simulink library "dotFinder_ul"  (R2018b)
settings: Solver=VariableStepAuto  StartTime=0.0  StopTime=10.0  RelTol=1e-3
libraries: simulink x2
settings Model: Creator=mcobb  LastModifiedBy=MAE-NCSUCORE
settings DebuggingCC: LibraryContextMissingDiagnostic=none
settings SFSimCC: SimUseLocalCustomCode=off
settings RTWCC: RTWUseLocalCustomCode=off

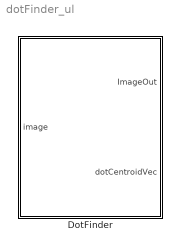
== system dotFinder_ul ==
  DotFinder : Subsystem  mask{ROIPositionHoldEnable=on, ROIPositionHoldCoordinates=[500 500], ROIDimVec_px=[30 90], ROIHalfDimVec_px=[15 45], ROISplitDims_px=[1 15 ; 1 90 ; 16 14 ; 1 90], DotOrientation=Vertical, OverlayOutput=on, ImageDimensions=[765 998], CrosshairPixelWidth_px=1}
      mask prompts: ROIPositionHoldEnable "Hold Position Enable"; ROIPositionHoldCoordinates "Hold Position Coordinates  [rows cols]  (pixels)"; ROIDimVec_px "Dimensions [rows cols]  (pixels)"; ROIHalfDimVec_px "Half Dims  [rows cols]  (pixels)"; ROISplitDims_px "Split Dims [rows cols]  (pixels)"; DotOrientation "Dot Orientation"; OverlayOutput "Draw Output Overlay"; ImageDimensions "Image Dimensions [rows cols] pixels"; CrosshairPixelWidth_px "Crosshair Width (pixels)"
      mask init:
      | dotFinder_init
      mask TypeOptions DotOrientation: Horizontal | Vertical
      mask DialogControl ParameterGroupVar Prompt: Region Of Interest (ROI) Parameters
      mask DialogControl Container3 Prompt: Other Parameters

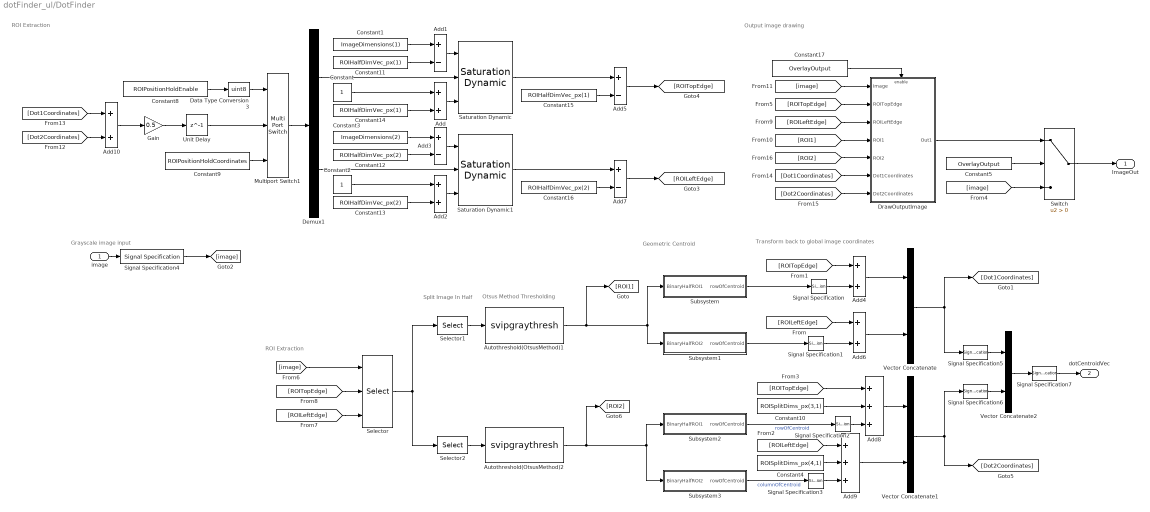
== system dotFinder_ul/DotFinder ==
  note: Transform back to global image coordinates
  note: Geometric Centroid
  note: Otsus Method Thresholding
  note: Split Image
      | In Half
  note: ROI Extraction
  note: Output image drawing
  note: ROI Extraction
  note: Grayscale image input
  image : Inport
  Add{,2,4,6,10} (5 alike) : Sum
  Add{1,3,5,7} (4 alike) : Sum  Inputs=+-
  Add8 : Sum  Inputs=+++
  Add9 : Sum  Inputs=+++
  Autothreshold(OtsusMethod)1 : S-Function  DialogController=vipDDGCreate  FunctionName=svipgraythresh  Parameters=operator, userDefinedRange, umin, umax, threshOut, effMetricOut, outOfRngOpt, scaleThreshold, scaleFactor, P1Mode, P1WordLength, P1FracLength, A1Mode, A1WordLength, A1FracLength, P2Mode, P2WordLength, P2FracLength, A2Mode, A2WordLength, A2FracLength, P3Mode, P3WordLength, P3FracLength, A3Mode, A3WordLength, A3FracLength, P4Mode, P4WordLength, P4FracLength, A4Mode, A4WordLength, A4FracLength, Q1Mode, Q1WordLength, Q1FracLength, EMMode, EMWordLength, EMFracLength, dtInfo.roundingMode, dtInfo.overflowMode  SFunctionDeploymentMode=off  EnableBusSupport=off  mask(Autothreshold){operator=>, threshOut=off, effMetricOut=off, userDefinedRange=off, umin=0, umax=255, outOfRngOpt=Ignore, scaleThreshold=off, scaleFactor=1, P1Mode=Specify word length, P1WordLength=32, P1FracLength=30, A1Mode=Same as Product 1, A1WordLength=32, A1FracLength=30, P2Mode=Specify word length, P2WordLength=32, P2FracLength=22, A2Mode=Same as Product 2, A2WordLength=32, A2FracLength=22, P3Mode=Specify word length, P3WordLength=32, P3FracLength=14, A3Mode=Same as Product 3, A3WordLength=32, A3FracLength=14, P4Mode=Binary point scaling, P4WordLength=32, P4FracLength=15, A4Mode=Same as Product 4, A4WordLength=16, A4FracLength=4, Q1Mode=Specify word length, Q1WordLength=32, Q1FracLength=16, EMMode=Specify word length, EMWordLength=16, EMFracLength=14, roundingMode=Floor, overflowMode=off, LockScale=off}
      mask prompts: operator "vision:masks:ThresholdingOperator"; threshOut "vision:masks:OutputThreshold"; effMetricOut "vision:masks:OutputEffectivenessMetric"; userDefinedRange "vision:masks:SpecifyDataRange"; umin "vision:masks:MinimumValueOfInput"; umax "vision:masks:MinimumValueOfInput"; outOfRngOpt "vision:masks:WhenDataRangeIsExceeded"; scaleThreshold "vision:masks:ScaleThreshold_MP"; scaleFactor "vision:masks:ThresholdScalingFactor"; P1Mode "P1:"; P1WordLength "P1 WL:"; P1FracLength "P1 FL:"; A1Mode "A1:"; A1WordLength "A1 WL:"; A1FracLength "A1 FL:"; P2Mode "P2:"; P2WordLength "P2 WL:"; P2FracLength "P2 FL:"; A2Mode "A2:"; A2WordLength "A2 WL:"; A2FracLength "A2 FL:"; P3Mode "P3:"; P3WordLength "P3 WL:"; P3FracLength "P3 FL:"; A3Mode "A3:"; A3WordLength "A3 WL:"; A3FracLength "A3 FL:"; P4Mode "P4:"; P4WordLength "P4 WL:"; P4FracLength "P4 FL:"; A4Mode "A4:"; A4WordLength "A4 WL:"; A4FracLength "A4 FL:"; Q1Mode "Q1:"; Q1WordLength "Q1 WL:"; Q1FracLength "Q1 FL:"; EMMode "EM:"; EMWordLength "EM WL:"; EMFracLength "EM FL:"; roundingMode "vision:masks:RoundIntegerCalculationsTowards"; overflowMode "vision:masks:RoundIntegerCalculationsTowards"; LockScale "vision:masks:LockScaling"
      mask help: vision:masks:AutoThresholdDescription
      mask init:
      | blk = gcbh;
      | 
      | dtInfo = dspGetFixptDataTypeInfo(blk,1);
      | 
      | effMetricOut_str = get_param(blk,'effMetricOut');
      | threshOut_str = get_param(blk,'threshOut');
      | if strcmp(effMetricOut_str,'off') && strcmp(threshOut_str,'off')
      | 	[so(1:3).port] = deal(1,1,1);
      | 	[so(1:3).txt] = deal('BW','BW','BW');
      | elseif strcmp(effMetricOut_str,'on') && strcmp(threshOut_str,'off')
      | 	[so(1:3).port] = deal(1,2,2);
      | 	[so(1:3).txt] = deal('BW','EMetric','EMetric');
      | elseif strcmp(effMetricOut_str,'off') && strcmp(threshOut_str,'on')
      | 	[so(1:3).port] = deal(1,2,2);
      | 	[so(1:3).txt] = deal('BW','Th','Th');
      | else
      | 	[so(1:3).port] = deal(1,2,3);
      | 	[so(1:3).txt] = deal('BW','Th','EMetric');
      | end
      mask Help: eval('visionblockhelp');
      mask TypeOptions operator: > | <=
      mask TypeOptions outOfRngOpt: vision:masks:Ignore | vision:masks:Saturate | vision:masks:WarnAndSaturate | vision:masks:Error
      mask TypeOptions P1Mode: Specify word length | Binary point scaling | Slope and bias scaling
      mask TypeOptions A1Mode: Same as Product 1 | Specify word length | Binary point scaling | Slope and bias scaling
      mask TypeOptions P2Mode: Specify word length | Binary point scaling | Slope and bias scaling
      mask TypeOptions A2Mode: Same as Product 2 | Specify word length | Binary point scaling | Slope and bias scaling
      mask TypeOptions P3Mode: Specify word length | Binary point scaling | Slope and bias scaling
      mask TypeOptions A3Mode: Same as Product 3 | Specify word length | Binary point scaling | Slope and bias scaling
      mask TypeOptions P4Mode: Same as input | Binary point scaling | Slope and bias scaling
      mask TypeOptions A4Mode: Same as Product 4 | Binary point scaling | Slope and bias scaling
      mask TypeOptions Q1Mode: Specify word length | Binary point scaling | Slope and bias scaling
      mask TypeOptions EMMode: Specify word length | Binary point scaling | Slope and bias scaling
      mask TypeOptions roundingMode: dspshared:FixptDialog:Ceiling_CB | dspshared:FixptDialog:Convergent_CB | dspshared:FixptDialog:Floor_CB | dspshared:FixptDialog:Nearest_CB | dspshared:FixptDialog:Round_CB | dspshared:FixptDialog:Simplest_CB | dspshared:FixptDialog:Zero_CB
      mask Display:
      | disp('Autothreshold');
      | port_label('input',1,'I');
      | port_label('output',so(1).port, so(1).txt);
      | port_label('output',so(2).port, so(2).txt);
      | port_label('output',so(3).port, so(3).txt);
  Autothreshold(OtsusMethod)2 : S-Function  DialogController=vipDDGCreate  FunctionName=svipgraythresh  Parameters=operator, userDefinedRange, umin, umax, threshOut, effMetricOut, outOfRngOpt, scaleThreshold, scaleFactor, P1Mode, P1WordLength, P1FracLength, A1Mode, A1WordLength, A1FracLength, P2Mode, P2WordLength, P2FracLength, A2Mode, A2WordLength, A2FracLength, P3Mode, P3WordLength, P3FracLength, A3Mode, A3WordLength, A3FracLength, P4Mode, P4WordLength, P4FracLength, A4Mode, A4WordLength, A4FracLength, Q1Mode, Q1WordLength, Q1FracLength, EMMode, EMWordLength, EMFracLength, dtInfo.roundingMode, dtInfo.overflowMode  SFunctionDeploymentMode=off  EnableBusSupport=off  mask(Autothreshold){operator=>, threshOut=off, effMetricOut=off, userDefinedRange=off, umin=0, umax=255, outOfRngOpt=Ignore, scaleThreshold=off, scaleFactor=1, P1Mode=Specify word length, P1WordLength=32, P1FracLength=30, A1Mode=Same as Product 1, A1WordLength=32, A1FracLength=30, P2Mode=Specify word length, P2WordLength=32, P2FracLength=22, A2Mode=Same as Product 2, A2WordLength=32, A2FracLength=22, P3Mode=Specify word length, P3WordLength=32, P3FracLength=14, A3Mode=Same as Product 3, A3WordLength=32, A3FracLength=14, P4Mode=Binary point scaling, P4WordLength=32, P4FracLength=15, A4Mode=Same as Product 4, A4WordLength=16, A4FracLength=4, Q1Mode=Specify word length, Q1WordLength=32, Q1FracLength=16, EMMode=Specify word length, EMWordLength=16, EMFracLength=14, roundingMode=Floor, overflowMode=off, LockScale=off}
      mask prompts: operator "vision:masks:ThresholdingOperator"; threshOut "vision:masks:OutputThreshold"; effMetricOut "vision:masks:OutputEffectivenessMetric"; userDefinedRange "vision:masks:SpecifyDataRange"; umin "vision:masks:MinimumValueOfInput"; umax "vision:masks:MinimumValueOfInput"; outOfRngOpt "vision:masks:WhenDataRangeIsExceeded"; scaleThreshold "vision:masks:ScaleThreshold_MP"; scaleFactor "vision:masks:ThresholdScalingFactor"; P1Mode "P1:"; P1WordLength "P1 WL:"; P1FracLength "P1 FL:"; A1Mode "A1:"; A1WordLength "A1 WL:"; A1FracLength "A1 FL:"; P2Mode "P2:"; P2WordLength "P2 WL:"; P2FracLength "P2 FL:"; A2Mode "A2:"; A2WordLength "A2 WL:"; A2FracLength "A2 FL:"; P3Mode "P3:"; P3WordLength "P3 WL:"; P3FracLength "P3 FL:"; A3Mode "A3:"; A3WordLength "A3 WL:"; A3FracLength "A3 FL:"; P4Mode "P4:"; P4WordLength "P4 WL:"; P4FracLength "P4 FL:"; A4Mode "A4:"; A4WordLength "A4 WL:"; A4FracLength "A4 FL:"; Q1Mode "Q1:"; Q1WordLength "Q1 WL:"; Q1FracLength "Q1 FL:"; EMMode "EM:"; EMWordLength "EM WL:"; EMFracLength "EM FL:"; roundingMode "vision:masks:RoundIntegerCalculationsTowards"; overflowMode "vision:masks:RoundIntegerCalculationsTowards"; LockScale "vision:masks:LockScaling"
      mask help: vision:masks:AutoThresholdDescription
      mask init: same as dotFinder_ul/DotFinder/Autothreshold(OtsusMethod)1
      mask Help: eval('visionblockhelp');
      mask TypeOptions operator: > | <=
      mask TypeOptions outOfRngOpt: vision:masks:Ignore | vision:masks:Saturate | vision:masks:WarnAndSaturate | vision:masks:Error
      mask TypeOptions P1Mode: Specify word length | Binary point scaling | Slope and bias scaling
      mask TypeOptions A1Mode: Same as Product 1 | Specify word length | Binary point scaling | Slope and bias scaling
      mask TypeOptions P2Mode: Specify word length | Binary point scaling | Slope and bias scaling
      mask TypeOptions A2Mode: Same as Product 2 | Specify word length | Binary point scaling | Slope and bias scaling
      mask TypeOptions P3Mode: Specify word length | Binary point scaling | Slope and bias scaling
      mask TypeOptions A3Mode: Same as Product 3 | Specify word length | Binary point scaling | Slope and bias scaling
      mask TypeOptions P4Mode: Same as input | Binary point scaling | Slope and bias scaling
      mask TypeOptions A4Mode: Same as Product 4 | Binary point scaling | Slope and bias scaling
      mask TypeOptions Q1Mode: Specify word length | Binary point scaling | Slope and bias scaling
      mask TypeOptions EMMode: Specify word length | Binary point scaling | Slope and bias scaling
      mask TypeOptions roundingMode: dspshared:FixptDialog:Ceiling_CB | dspshared:FixptDialog:Convergent_CB | dspshared:FixptDialog:Floor_CB | dspshared:FixptDialog:Nearest_CB | dspshared:FixptDialog:Round_CB | dspshared:FixptDialog:Simplest_CB | dspshared:FixptDialog:Zero_CB
      mask Display:
      | disp('Autothreshold');
      | port_label('input',1,'I');
      | port_label('output',so(1).port, so(1).txt);
      | port_label('output',so(2).port, so(2).txt);
      | port_label('output',so(3).port, so(3).txt);
  Constant : Constant
  Constant1 : Constant  Value=ImageDimensions(1)
  Constant10 : Constant  Value=ROISplitDims_px(3,1)
  Constant11 : Constant  Value=ROIHalfDimVec_px(1)
  Constant12 : Constant  Value=ROIHalfDimVec_px(2)
  Constant13 : Constant  Value=ROIHalfDimVec_px(2)
  Constant14 : Constant  Value=ROIHalfDimVec_px(1)
  Constant15 : Constant  Value=ROIHalfDimVec_px(1)
  Constant16 : Constant  Value=ROIHalfDimVec_px(2)
  Constant17 : Constant  Value=OverlayOutput
  Constant2 : Constant
  Constant3 : Constant  Value=ImageDimensions(2)
  Constant4 : Constant  Value=ROISplitDims_px(4,1)
  Constant5 : Constant  Value=OverlayOutput
  Constant8 : Constant  Value=ROIPositionHoldEnable
  Constant9 : Constant  Value=ROIPositionHoldCoordinates
  Data Type Conversion3 : DataTypeConversion  OutDataTypeStr=uint8
  Demux1 : Demux  Outputs=2
  DrawOutputImage : Subsystem
  Gain : Gain  Gain=0.5
  Multiport Switch1 : MultiPortSwitch  DataPortOrder=Zero-based contiguous  Inputs=2  zeroidx=on
  Saturation Dynamic : simulink/Discontinuities/Saturation Dynamic  OutMin=[]  OutMax=[]  OutDataTypeStr=Inherit: Same as second input  OutDataType=fixdt(1, 16)  OutScaling=2^-10  DoSatur=off
  Saturation Dynamic1 : simulink/Discontinuities/Saturation Dynamic  OutMin=[]  OutMax=[]  OutDataTypeStr=Inherit: Same as second input  OutDataType=fixdt(1, 16)  OutScaling=2^-10  DoSatur=off
  Selector : Selector  NumberOfDimensions=2  InputPortWidth=3  IndexOptions=Starting index (port),Starting index (port)  Indices=[1 3],1  OutputSizes=ROIDimVec_px(1),ROIDimVec_px(2)
  Selector1 : Selector  NumberOfDimensions=2  InputPortWidth=3  IndexOptions=Starting index (dialog),Starting index (dialog)  Indices=ROISplitDims_px(1,1),ROISplitDims_px(2,1)  OutputSizes=ROISplitDims_px(1,2),ROISplitDims_px(2,2)
  Selector2 : Selector  NumberOfDimensions=2  InputPortWidth=3  IndexOptions=Starting index (dialog),Starting index (dialog)  Indices=ROISplitDims_px(3,1),ROISplitDims_px(4,1)  OutputSizes=ROISplitDims_px(3,2),ROISplitDims_px(4,2)
  Signal Specification{,1..3} (4 alike) : SignalSpecification  Dimensions=1
  Signal Specification4 : SignalSpecification  Dimensions=ImageDimensions
  Signal Specification5 : SignalSpecification  Dimensions=[1 2]
  Signal Specification6 : SignalSpecification  Dimensions=[1 2]
  Signal Specification7 : SignalSpecification  Dimensions=[1 4]
  Subsystem : Subsystem
  Subsystem1 : Subsystem
  Subsystem2 : Subsystem
  Subsystem3 : Subsystem
  Switch : Switch  Criteria=u2 > Threshold
  Unit Delay : Delay  DelayLength=1  InitialCondition=ROIPositionHoldCoordinates
  Vector Concatenate : Concatenate
  Vector Concatenate1 : Concatenate
  Vector Concatenate2 : Concatenate  ConcatenateDimension=2
  ImageOut : Outport  PortDimensions=ImageDimensions
  dotCentroidVec : Outport  Port=2
  wires:
  Data Type Conversion3/1 -> Multiport Switch1/1
  Unit Delay/1 -> Multiport Switch1/2
  Multiport Switch1/1 -> Demux1/1
  Demux1/1 -> Saturation Dynamic/2
  Constant/1 -> Add/1
  Constant14/1 -> Add/2
  Constant1/1 -> Add1/1
  Constant11/1 -> Add1/2
  Constant12/1 -> Add3/2
  Constant3/1 -> Add3/1
  Constant13/1 -> Add2/2
  Constant2/1 -> Add2/1
  Demux1/2 -> Saturation Dynamic1/2
  Constant15/1 -> Add5/2
  Constant16/1 -> Add7/2
  [image] -> Selector/1
  Selector/1 -> Selector2/1, Selector1/1
  Constant8/1 -> Data Type Conversion3/1
  Constant9/1 -> Multiport Switch1/3
  Saturation Dynamic/1 -> Add5/1
  Saturation Dynamic1/1 -> Add7/1
  Add2/1 -> Saturation Dynamic1/3
  Add3/1 -> Saturation Dynamic1/1
  Add/1 -> Saturation Dynamic/3
  Add1/1 -> Saturation Dynamic/1
  Subsystem1/1(rowOfCentroid) -> Signal Specification1/1
  [ROITopEdge] -> Add4/1
  [ROILeftEdge] -> Add6/1
  Add4/1 -> Vector Concatenate/1
  Add6/1 -> Vector Concatenate/2
  Add9/1 -> Vector Concatenate1/2
  Add8/1 -> Vector Concatenate1/1
  [ROILeftEdge] -> Add9/1
  [ROITopEdge] -> Add8/1
  Subsystem3/1(rowOfCentroid) -> Signal Specification3/1  "columnOfCentroid"
  Subsystem2/1(rowOfCentroid) -> Signal Specification2/1  "rowOfCentroid"
  Selector2/1 -> Autothreshold(OtsusMethod)2/1
  Constant4/1 -> Add9/2
  Constant10/1 -> Add8/2
  Vector Concatenate1/1 -> Signal Specification6/1, [Dot2Coordinates]
  image/1 -> Signal Specification4/1
  Add7/1 -> [ROILeftEdge]
  Add5/1 -> [ROITopEdge]
  Constant17/1 -> DrawOutputImage/Enable
  DrawOutputImage/1(Out1) -> Switch/1
  [ROILeftEdge] -> Selector/3
  [ROITopEdge] -> Selector/2
  [ROITopEdge] -> DrawOutputImage/2(ROITopEdge)
  [ROILeftEdge] -> DrawOutputImage/3(ROILeftEdge)
  [ROI1] -> DrawOutputImage/4(ROI1)
  [image] -> Switch/3
  Constant5/1 -> Switch/2
  [image] -> DrawOutputImage/1(Image)
  Vector Concatenate/1 -> Signal Specification5/1, [Dot1Coordinates]
  [Dot2Coordinates] -> DrawOutputImage/7(Dot2Coordinates)
  [Dot1Coordinates] -> DrawOutputImage/6(Dot1Coordinates)
  Switch/1 -> ImageOut/1
  Selector1/1 -> Autothreshold(OtsusMethod)1/1
  Signal Specification/1 -> Add4/2
  Signal Specification1/1 -> Add6/2
  Signal Specification2/1 -> Add8/3
  Signal Specification3/1 -> Add9/3
  Signal Specification4/1 -> [image]
  Subsystem/1(rowOfCentroid) -> Signal Specification/1
  Autothreshold(OtsusMethod)2/1 -> [ROI2], Subsystem3/1(BinaryHalfROI2), Subsystem2/1(BinaryHalfROI1)
  Autothreshold(OtsusMethod)1/1 -> [ROI1], Subsystem1/1(BinaryHalfROI2), Subsystem/1(BinaryHalfROI1)
  [ROI2] -> DrawOutputImage/5(ROI2)
  Add10/1 -> Gain/1
  [Dot2Coordinates] -> Add10/2
  [Dot1Coordinates] -> Add10/1
  Gain/1 -> Unit Delay/1
  Vector Concatenate2/1 -> Signal Specification7/1
  Signal Specification5/1 -> Vector Concatenate2/1
  Signal Specification6/1 -> Vector Concatenate2/2
  Signal Specification7/1 -> dotCentroidVec/1

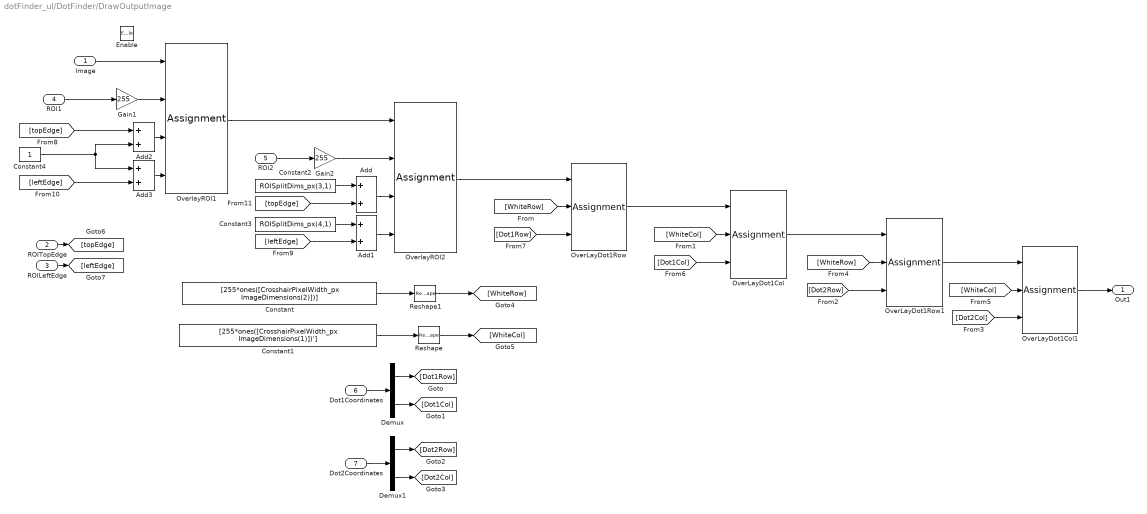
== system dotFinder_ul/DotFinder/DrawOutputImage ==
  Image : Inport
  ROITopEdge : Inport  Port=2
  ROILeftEdge : Inport  Port=3
  ROI1 : Inport  Port=4
  ROI2 : Inport  Port=5
  Dot1Coordinates : Inport  Port=6  PortDimensions=2
  Dot2Coordinates : Inport  Port=7  PortDimensions=2
  Enable : EnablePort
  Add{,1..3} (4 alike) : Sum
  Constant : Constant  Value=[255*ones([CrosshairPixelWidth_px ImageDimensions(2)])]  OutDataTypeStr=uint8
  Constant1 : Constant  Value=[255*ones([CrosshairPixelWidth_px ImageDimensions(1)])']  OutDataTypeStr=uint8
  Constant2 : Constant  Value=ROISplitDims_px(3,1)
  Constant3 : Constant  Value=ROISplitDims_px(4,1)
  Constant4 : Constant
  Demux : Demux  Outputs=2
  Demux1 : Demux  Outputs=2
  Gain1 : Gain  Gain=255  OutDataTypeStr=uint8
  Gain2 : Gain  Gain=255  OutDataTypeStr=uint8
  OverLayDot1Col : Assignment  NumberOfDimensions=2  DiagnosticForDimensions=Warning  IndexOptions=Assign all,Starting index (port)  Indices=1,1  OutputSizes=1,1
  OverLayDot1Col1 : Assignment  NumberOfDimensions=2  DiagnosticForDimensions=Warning  IndexOptions=Assign all,Starting index (port)  Indices=1,1  OutputSizes=1,1
  OverLayDot1Row : Assignment  NumberOfDimensions=2  DiagnosticForDimensions=Warning  IndexOptions=Starting index (port),Assign all  Indices=1,1  OutputSizes=1,1
  OverLayDot1Row1 : Assignment  NumberOfDimensions=2  DiagnosticForDimensions=Warning  IndexOptions=Starting index (port),Assign all  Indices=1,1  OutputSizes=1,1
  OverlayROI1 : Assignment  NumberOfDimensions=2  DiagnosticForDimensions=Warning  IndexOptions=Starting index (port),Starting index (port)  Indices=1,1  OutputSizes=1,1
  OverlayROI2 : Assignment  NumberOfDimensions=2  DiagnosticForDimensions=Warning  IndexOptions=Starting index (port),Starting index (port)  Indices=1,1  OutputSizes=1,1
  Reshape : Reshape  OutputDimensionality=Customize  OutputDimensions=[ImageDimensions(1) CrosshairPixelWidth_px ]
  Reshape1 : Reshape  OutputDimensionality=Customize  OutputDimensions=[CrosshairPixelWidth_px ImageDimensions(2)]
  Out1 : Outport
  wires:
  Gain1/1 -> OverlayROI1/2
  Image/1 -> OverlayROI1/1
  Dot1Coordinates/1 -> Demux/1
  Dot2Coordinates/1 -> Demux1/1
  Demux/1 -> [Dot1Row]
  Demux/2 -> [Dot1Col]
  Demux1/1 -> [Dot2Row]
  Demux1/2 -> [Dot2Col]
  Constant/1 -> Reshape1/1
  Constant1/1 -> Reshape/1
  OverLayDot1Row/1 -> OverLayDot1Col/1
  OverLayDot1Col/1 -> OverLayDot1Row1/1
  OverLayDot1Row1/1 -> OverLayDot1Col1/1
  [WhiteRow] -> OverLayDot1Row/2
  [WhiteCol] -> OverLayDot1Col/2
  [Dot2Row] -> OverLayDot1Row1/3
  [Dot2Col] -> OverLayDot1Col1/3
  [WhiteRow] -> OverLayDot1Row1/2
  [WhiteCol] -> OverLayDot1Col1/2
  [Dot1Col] -> OverLayDot1Col/3
  [Dot1Row] -> OverLayDot1Row/3
  Reshape1/1 -> [WhiteRow]
  Reshape/1 -> [WhiteCol]
  OverlayROI1/1 -> OverlayROI2/1
  Gain2/1 -> OverlayROI2/2
  Add/1 -> OverlayROI2/3
  Add1/1 -> OverlayROI2/4
  Constant2/1 -> Add/1
  Constant3/1 -> Add1/1
  ROITopEdge/1 -> [topEdge]
  ROILeftEdge/1 -> [leftEdge]
  [leftEdge] -> Add1/2
  [topEdge] -> Add/2
  OverlayROI2/1 -> OverLayDot1Row/1
  Add2/1 -> OverlayROI1/3
  Add3/1 -> OverlayROI1/4
  [topEdge] -> Add2/1
  [leftEdge] -> Add3/2
  Constant4/1 -> Add3/1, Add2/2
  OverLayDot1Col1/1 -> Out1/1
  ROI2/1 -> Gain2/1
  ROI1/1 -> Gain1/1

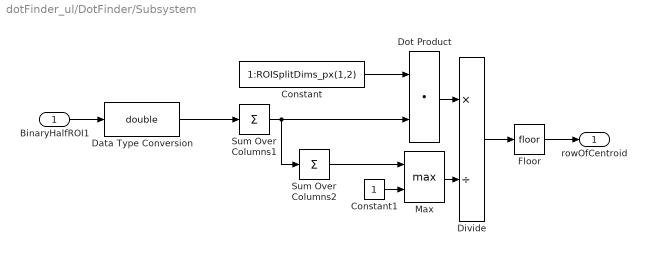
== system dotFinder_ul/DotFinder/Subsystem ==
  BinaryHalfROI1 : Inport
  Constant : Constant  Value=1:ROISplitDims_px(1,2)
  Constant1 : Constant
  Data Type Conversion : DataTypeConversion  OutDataTypeStr=double
  Divide : Product  Inputs=*/
  Dot Product : DotProduct  InputSameDT=on  OutDataTypeStr=Inherit: Inherit via internal rule
  Floor : Rounding
  Max : MinMax  Function=max  Inputs=2
  Sum Over Columns1 : Sum  Inputs=+  CollapseMode=Specified dimension  CollapseDim=2
  Sum Over Columns2 : Sum  Inputs=+  CollapseDim=2
  rowOfCentroid : Outport
  wires:
  BinaryHalfROI1/1 -> Data Type Conversion/1
  Divide/1 -> Floor/1
  Constant/1 -> Dot Product/1
  Dot Product/1 -> Divide/1
  Sum Over Columns1/1 -> Sum Over Columns2/1, Dot Product/2
  Sum Over Columns2/1 -> Max/1
  Max/1 -> Divide/2
  Constant1/1 -> Max/2
  Floor/1 -> rowOfCentroid/1
  Data Type Conversion/1 -> Sum Over Columns1/1

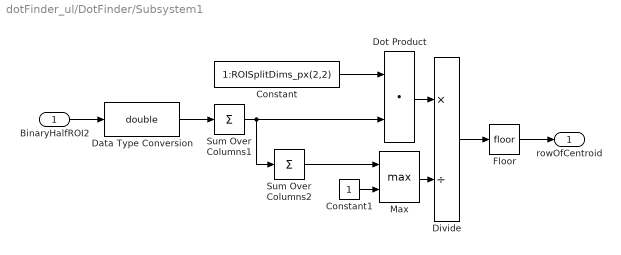
== system dotFinder_ul/DotFinder/Subsystem1 ==
  BinaryHalfROI2 : Inport
  Constant : Constant  Value=1:ROISplitDims_px(2,2)
  Constant1 : Constant
  Data Type Conversion : DataTypeConversion  OutDataTypeStr=double
  Divide : Product  Inputs=*/
  Dot Product : DotProduct  InputSameDT=on  OutDataTypeStr=Inherit: Inherit via internal rule
  Floor : Rounding
  Max : MinMax  Function=max  Inputs=2
  Sum Over Columns1 : Sum  Inputs=+  CollapseMode=Specified dimension
  Sum Over Columns2 : Sum  Inputs=+  CollapseDim=2
  rowOfCentroid : Outport
  wires:
  Floor/1 -> rowOfCentroid/1
  Constant1/1 -> Max/2
  Max/1 -> Divide/2
  Sum Over Columns2/1 -> Max/1
  Sum Over Columns1/1 -> Dot Product/2, Sum Over Columns2/1
  Dot Product/1 -> Divide/1
  Constant/1 -> Dot Product/1
  Divide/1 -> Floor/1
  BinaryHalfROI2/1 -> Data Type Conversion/1
  Data Type Conversion/1 -> Sum Over Columns1/1

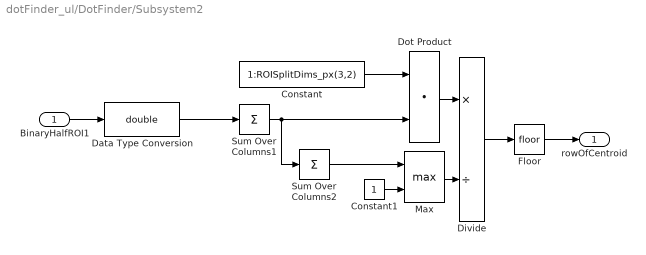
== system dotFinder_ul/DotFinder/Subsystem2 ==
  BinaryHalfROI1 : Inport
  Constant : Constant  Value=1:ROISplitDims_px(3,2)
  Constant1 : Constant
  Data Type Conversion : DataTypeConversion  OutDataTypeStr=double
  Divide : Product  Inputs=*/
  Dot Product : DotProduct  InputSameDT=on  OutDataTypeStr=Inherit: Inherit via internal rule
  Floor : Rounding
  Max : MinMax  Function=max  Inputs=2
  Sum Over Columns1 : Sum  Inputs=+  CollapseMode=Specified dimension  CollapseDim=2
  Sum Over Columns2 : Sum  Inputs=+  CollapseDim=2
  rowOfCentroid : Outport
  wires:
  Data Type Conversion/1 -> Sum Over Columns1/1
  Floor/1 -> rowOfCentroid/1
  Constant1/1 -> Max/2
  Max/1 -> Divide/2
  Sum Over Columns2/1 -> Max/1
  Sum Over Columns1/1 -> Dot Product/2, Sum Over Columns2/1
  Dot Product/1 -> Divide/1
  Constant/1 -> Dot Product/1
  Divide/1 -> Floor/1
  BinaryHalfROI1/1 -> Data Type Conversion/1

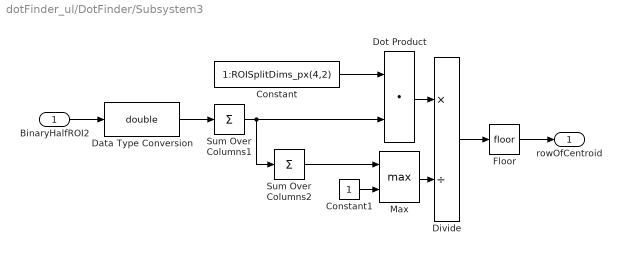
== system dotFinder_ul/DotFinder/Subsystem3 ==
  BinaryHalfROI2 : Inport
  Constant : Constant  Value=1:ROISplitDims_px(4,2)
  Constant1 : Constant
  Data Type Conversion : DataTypeConversion  OutDataTypeStr=double
  Divide : Product  Inputs=*/
  Dot Product : DotProduct  InputSameDT=on  OutDataTypeStr=Inherit: Inherit via internal rule
  Floor : Rounding
  Max : MinMax  Function=max  Inputs=2
  Sum Over Columns1 : Sum  Inputs=+  CollapseMode=Specified dimension
  Sum Over Columns2 : Sum  Inputs=+  CollapseDim=2
  rowOfCentroid : Outport
  wires:
  Data Type Conversion/1 -> Sum Over Columns1/1
  BinaryHalfROI2/1 -> Data Type Conversion/1
  Divide/1 -> Floor/1
  Constant/1 -> Dot Product/1
  Dot Product/1 -> Divide/1
  Sum Over Columns1/1 -> Sum Over Columns2/1, Dot Product/2
  Sum Over Columns2/1 -> Max/1
  Max/1 -> Divide/2
  Constant1/1 -> Max/2
  Floor/1 -> rowOfCentroid/1
